simulink library "eltreclib"  (R2017a)
settings: Solver=VariableStepAuto  StartTime=0.0  StopTime=10.0  RelTol=1e-3
libraries: powerlib x46
settings Model: Creator=mayartmal  LastModifiedBy=OspanbekovBK

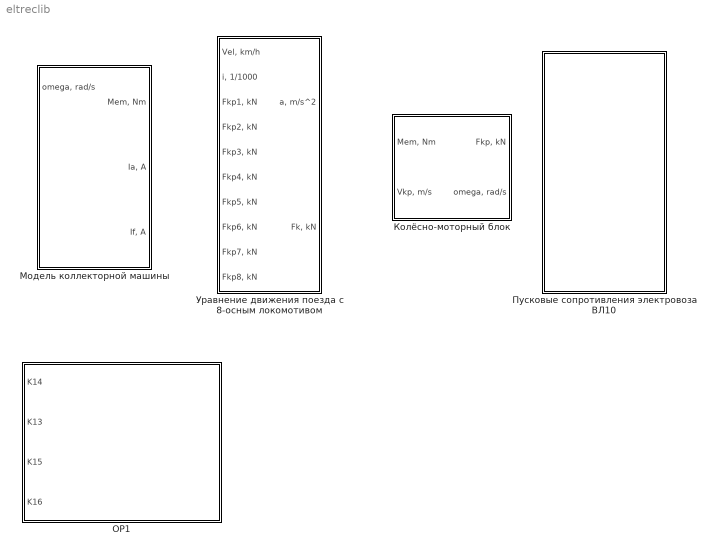
== system eltreclib ==
  OP1 : Subsystem
      mask DialogControl DescTextVar Prompt: Резисторы ослабления поля
  Колёсно-моторный блок : Subsystem  mask{Db=0, mu=0}
      mask prompts: Db "Диаметр бандажа, м"; mu "Передаточное отношение редуктора"
      mask DialogControl DescTextVar Prompt: Здесь можно вписать описание, формулы и другую полезную информацию
  Модель коллекторной машины : Subsystem  mask{Rf=0, Lf=0, Ra=0, La=0, Ce=0, Cm=0, A=0, B=0}
      mask prompts: Rf "Активное сопротивление обмотки возбуждения, Ом"; Lf "Индуктивность обмотки возбуждения, Гн"; Ra "Активное сопротивление обмотки якоря, Ом"; La "Индуктивность обмотки якоря, Гн"; Ce "Константа Ce"; Cm "Константа Cm"; A "Коэффициент A"; B "Коэффициент B"
      mask DialogControl DescTextVar Prompt: Здесь можно вписать описание, формулы и другую полезную информацию
  Пусковые сопротивления электровоза ВЛ10 : Subsystem
  Уравнение движения поезда c 8-осным локомотивом : Subsystem  mask{a0=0, a1=0, a2=0, P=0, Q=0}
      mask prompts: a0 "Коэффициент a0"; a1 "Коэффициент a1"; a2 "Коэффициент a2"; P "Масса локомотива, т"; Q "Масса состава, т"
      mask DialogControl DescTextVar Prompt: Здесь можно вписать описание, формулы и другую полезную информацию

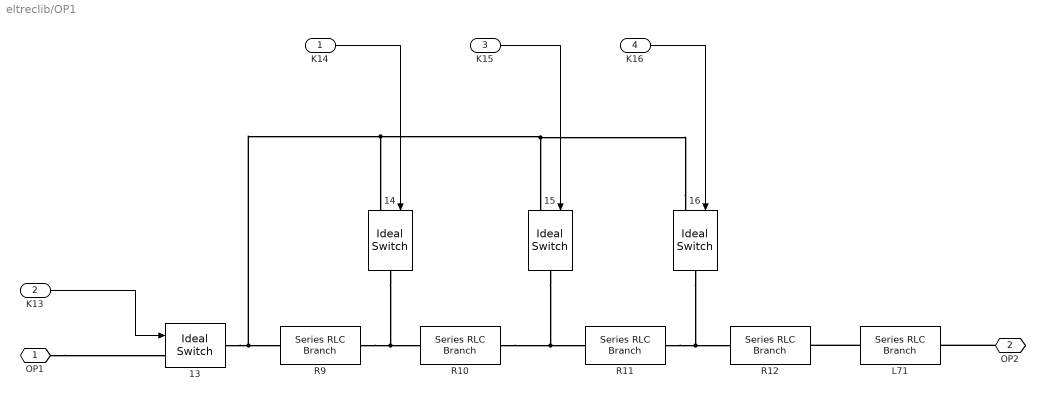
== system eltreclib/OP1 ==
  K14 : Inport
  K13 : Inport  Port=2
  K15 : Inport  Port=3
  K16 : Inport  Port=4
  {13..16} (4 alike) : powerlib/Power Electronics/Ideal Switch  Ron=0.001  Lon=0  IC=0  Rs=1e6  Cs=inf  Measurements=off
  L71 : powerlib/Elements/Series RLC Branch  LConnTagsString=__new0  RConnTagsString=__new0  BranchType=RL  Resistance=0.0236  Inductance=4.5e-3  SetiL0=off  InitialCurrent=0  Capacitance=1e-6  Setx0=off  InitialVoltage=0  Measurements=None
  R10 : powerlib/Elements/Series RLC Branch  LConnTagsString=__new0  RConnTagsString=__new0  BranchType=R  Resistance=0.04  Inductance=1e-3  SetiL0=off  InitialCurrent=0  Capacitance=1e-6  Setx0=off  InitialVoltage=0  Measurements=None
  R11 : powerlib/Elements/Series RLC Branch  LConnTagsString=__new0  RConnTagsString=__new0  BranchType=R  Resistance=0.0222  Inductance=1e-3  SetiL0=off  InitialCurrent=0  Capacitance=1e-6  Setx0=off  InitialVoltage=0  Measurements=None
  R12 : powerlib/Elements/Series RLC Branch  LConnTagsString=__new0  RConnTagsString=__new0  BranchType=R  Resistance=0.01  Inductance=1e-3  SetiL0=off  InitialCurrent=0  Capacitance=1e-6  Setx0=off  InitialVoltage=0  Measurements=None
  R9 : powerlib/Elements/Series RLC Branch  LConnTagsString=__new0  RConnTagsString=__new0  BranchType=R  Resistance=0.1407  Inductance=1e-3  SetiL0=off  InitialCurrent=0  Capacitance=1e-6  Setx0=off  InitialVoltage=0  Measurements=None
  OP1 : PMIOPort  Port=1  Side=Right
  OP2 : PMIOPort  Port=2  Side=Right
  wires:
  K16/1 -> 16/1
  K15/1 -> 15/1
  K13/1 -> 13/1
  K14/1 -> 14/1
  connections:
  OP2/RConn1 -- L71/RConn1
  L71/LConn1 -- R12/RConn1
  OP1/RConn1 -- 13/LConn1
  16/LConn1 -- 14/LConn1 -- 13/RConn1 -- R9/LConn1 -- 15/LConn1
  16/RConn1 -- R11/RConn1 -- R12/LConn1
  15/RConn1 -- R10/RConn1 -- R11/LConn1
  14/RConn1 -- R9/RConn1 -- R10/LConn1

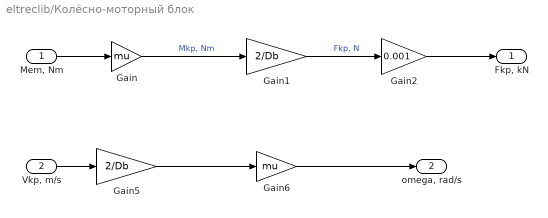
== system eltreclib/Колёсно-моторный блок ==
  "Mem, Nm" : Inport
  "Vkp, m/s" : Inport  Port=2
  Gain : Gain  Gain=mu
  Gain1 : Gain  Gain=2/Db
  Gain2 : Gain  Gain=0.001
  Gain5 : Gain  Gain=2/Db
  Gain6 : Gain  Gain=mu
  "Fkp, kN" : Outport
  "omega, rad/s" : Outport  Port=2
  wires:
  Gain/1 -> Gain1/1  "Mkp, Nm"
  "Mem, Nm"/1 -> Gain/1
  Gain1/1 -> Gain2/1  "Fkp, N"
  Gain5/1 -> Gain6/1
  "Vkp, m/s"/1 -> Gain5/1
  Gain6/1 -> "omega, rad/s"/1
  Gain2/1 -> "Fkp, kN"/1

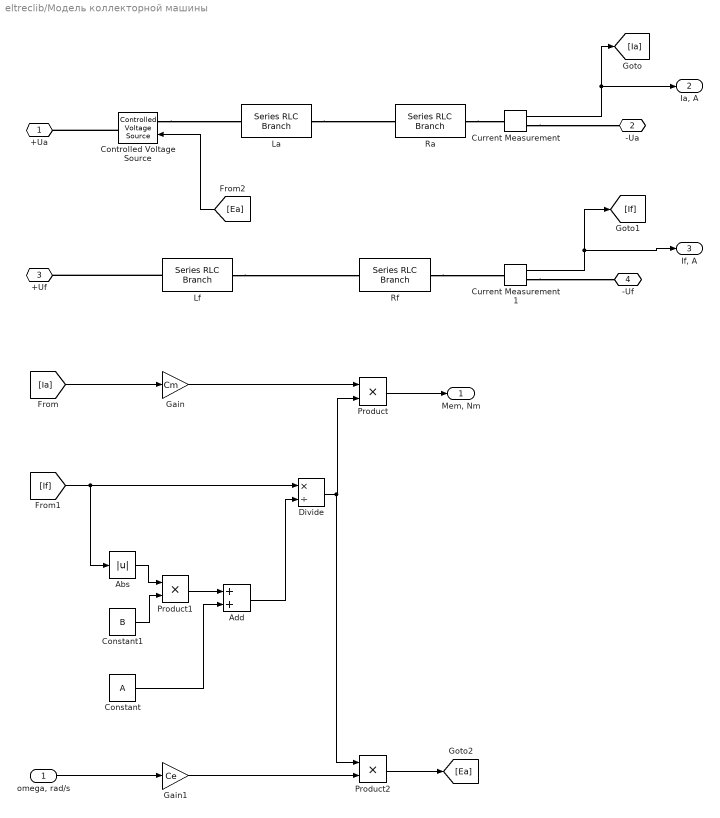
== system eltreclib/Модель коллекторной машины ==
  "omega, rad/s" : Inport
  Abs : Abs
  Add : Sum
  Constant : Constant  Value=A
  Constant1 : Constant  Value=B
  Controlled Voltage Source : powerlib/Electrical Sources/Controlled Voltage Source  Initialize=on  Source_Type=AC  Amplitude=0  Phase=0  Frequency=0  Measurements=None
  Current Measurement : powerlib/Measurements/Current Measurement  PhasorSimulation=off  OutputType=Complex  PSBequivalent=0
  Current Measurement1 : powerlib/Measurements/Current Measurement  PhasorSimulation=off  OutputType=Complex  PSBequivalent=0
  Divide : Product  Inputs=*/
  Gain : Gain  Gain=Cm
  Gain1 : Gain  Gain=Ce
  La : powerlib/Elements/Series RLC Branch  LConnTagsString=__new0  RConnTagsString=__new0  BranchType=L  Resistance=1  Inductance=La  SetiL0=off  InitialCurrent=0  Capacitance=1e-6  Setx0=off  InitialVoltage=0  Measurements=None
  Lf : powerlib/Elements/Series RLC Branch  LConnTagsString=__new0  RConnTagsString=__new0  BranchType=L  Resistance=1  Inductance=Lf  SetiL0=off  InitialCurrent=0  Capacitance=1e-6  Setx0=off  InitialVoltage=0  Measurements=None
  Product : Product
  Product1 : Product
  Product2 : Product
  Ra : powerlib/Elements/Series RLC Branch  LConnTagsString=__new0  RConnTagsString=__new0  BranchType=R  Resistance=Ra  Inductance=1e-3  SetiL0=off  InitialCurrent=0  Capacitance=1e-6  Setx0=off  InitialVoltage=0  Measurements=None
  Rf : powerlib/Elements/Series RLC Branch  LConnTagsString=__new0  RConnTagsString=__new0  BranchType=R  Resistance=Rf  Inductance=1e-3  SetiL0=off  InitialCurrent=0  Capacitance=1e-6  Setx0=off  InitialVoltage=0  Measurements=None
  +Ua : PMIOPort  Port=1  Side=Left
  -Ua : PMIOPort  Port=2  Side=Left
  +Uf : PMIOPort  Port=3  Side=Left
  -Uf : PMIOPort  Port=4  Side=Left
  "Mem, Nm" : Outport
  "Ia, A" : Outport  Port=2
  "If, A" : Outport  Port=3
  wires:
  Product/1 -> "Mem, Nm"/1
  Product2/1 -> [Ea]
  Gain1/1 -> Product2/2
  "omega, rad/s"/1 -> Gain1/1
  Divide/1 -> Product/2, Product2/1
  Add/1 -> Divide/2
  Product1/1 -> Add/1
  Constant/1 -> Add/2
  Constant1/1 -> Product1/2
  Abs/1 -> Product1/1
  [If] -> Abs/1, Divide/1
  Gain/1 -> Product/1
  [Ia] -> Gain/1
  Current Measurement1/1 -> [If], "If, A"/1
  Current Measurement/1 -> "Ia, A"/1, [Ia]
  [Ea] -> Controlled Voltage Source/1
  connections:
  Current Measurement1/RConn1 -- -Uf/RConn1
  Rf/RConn1 -- Current Measurement1/LConn1
  Current Measurement/RConn1 -- -Ua/RConn1
  Ra/RConn1 -- Current Measurement/LConn1
  Controlled Voltage Source/LConn1 -- La/LConn1
  Lf/RConn1 -- Rf/LConn1
  Controlled Voltage Source/RConn1 -- +Ua/RConn1
  Lf/LConn1 -- +Uf/RConn1
  La/RConn1 -- Ra/LConn1

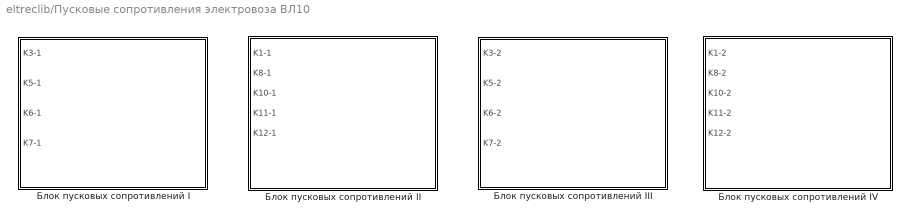
== system eltreclib/Пусковые сопротивления электровоза ВЛ10 ==
  Блок пусковых сопротивлений I : Subsystem
      mask DialogControl DescGroupVar Prompt: Блок пусковых сопротивлений I
      mask DialogControl DescTextVar Prompt: Моделирует схему блока пусковых сопротивлений, собранного из резисторов R1=3.15 Ом, R2=1.47 Ом, R3=1.2 Ом
  Блок пусковых сопротивлений II : Subsystem
      mask DialogControl DescGroupVar Prompt: Блок пусковых сопротивлений II
      mask DialogControl DescTextVar Prompt: Моделирует схему блока пусковых сопротивлений, собранного из резисторов R5=4.725 Ом, R6=0.841 Ом, R7=1.312 Ом
  Блок пусковых сопротивлений III : Subsystem
      mask DialogControl DescGroupVar Prompt: Блок пусковых сопротивлений III
      mask DialogControl DescTextVar Prompt: Моделирует схему блока пусковых сопротивлений, собранного из резисторов R23=1.9425 Ом, R24=0.8 Ом, R25=0.61 Ом
  Блок пусковых сопротивлений IV : Subsystem
      mask DialogControl DescGroupVar Prompt: Блок пусковых сопротивлений IV
      mask DialogControl DescTextVar Prompt: Моделирует схему блока пусковых сопротивлений, собранного из резисторов R27=5.775 Ом, R28=0.595 Ом, R29=0.4315 Ом

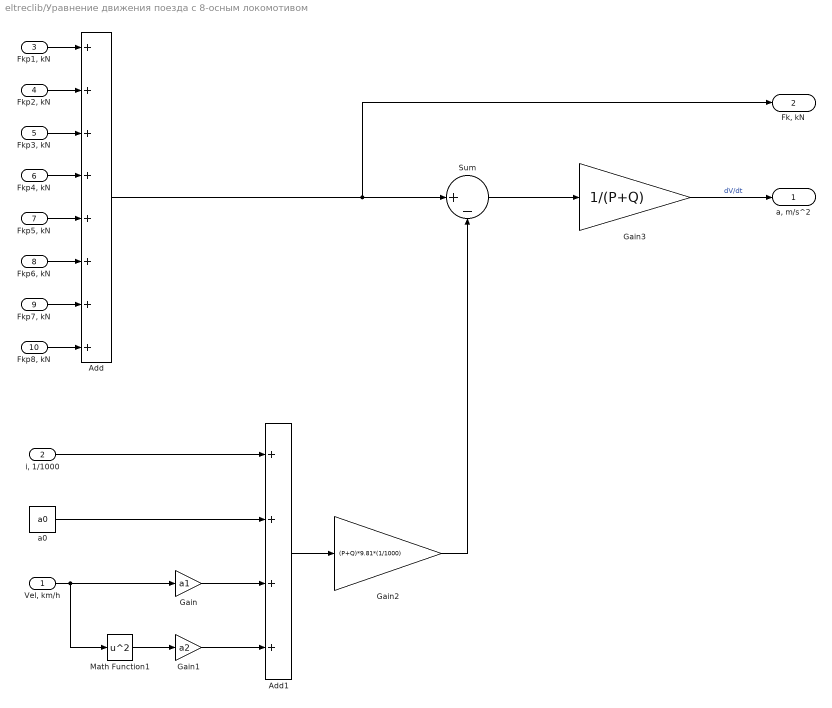
== system eltreclib/Уравнение движения поезда c 8-осным локомотивом ==
  "Vel, km/h" : Inport
  "i, 1/1000" : Inport  Port=2
  "Fkp1, kN" : Inport  Port=3
  "Fkp2, kN" : Inport  Port=4
  "Fkp3, kN" : Inport  Port=5
  "Fkp4, kN" : Inport  Port=6
  "Fkp5, kN" : Inport  Port=7
  "Fkp6, kN" : Inport  Port=8
  "Fkp7, kN" : Inport  Port=9
  "Fkp8, kN" : Inport  Port=10
  Add : Sum  Inputs=++++++++
  Add1 : Sum  Inputs=++++
  Gain : Gain  Gain=a1
  Gain1 : Gain  Gain=a2
  Gain2 : Gain  Gain=(P+Q)*9.81*(1/1000)
  Gain3 : Gain  Gain=1/(P+Q)
  Math Function1 : Math  Operator=square  SaturateOnIntegerOverflow=on
  Sum : Sum  Inputs=|+-
  a0 : Constant  Value=a0
  "a, m/s^2" : Outport
  "Fk, kN" : Outport  Port=2
  wires:
  Add/1 -> "Fk, kN"/1, Sum/1
  "Vel, km/h"/1 -> Math Function1/1, Gain/1
  a0/1 -> Add1/2
  Gain/1 -> Add1/3
  Sum/1 -> Gain3/1
  Gain3/1 -> "a, m/s^2"/1  "dV/dt"
  Gain2/1 -> Sum/2
  Math Function1/1 -> Gain1/1
  Gain1/1 -> Add1/4
  Add1/1 -> Gain2/1
  "Fkp7, kN"/1 -> Add/7
  "Fkp4, kN"/1 -> Add/4
  "Fkp8, kN"/1 -> Add/8
  "Fkp5, kN"/1 -> Add/5
  "Fkp6, kN"/1 -> Add/6
  "Fkp1, kN"/1 -> Add/1
  "Fkp3, kN"/1 -> Add/3
  "Fkp2, kN"/1 -> Add/2
  "i, 1/1000"/1 -> Add1/1

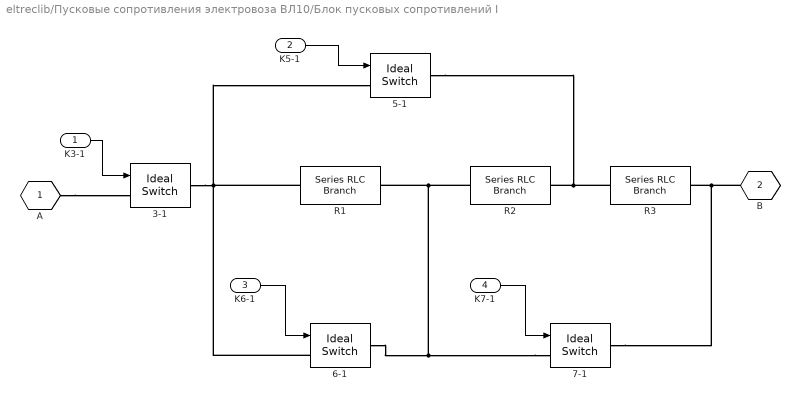
== system eltreclib/Пусковые сопротивления электровоза ВЛ10/Блок пусковых сопротивлений I ==
  K3-1 : Inport
  K5-1 : Inport  Port=2
  K6-1 : Inport  Port=3
  K7-1 : Inport  Port=4
  3-1 : powerlib/Power Electronics/Ideal Switch  Ron=0.001  Lon=0  IC=0  Rs=1e6  Cs=inf  Measurements=off
  5-1 : powerlib/Power Electronics/Ideal Switch  Ron=0.001  Lon=0  IC=0  Rs=1e6  Cs=inf  Measurements=off
  6-1 : powerlib/Power Electronics/Ideal Switch  Ron=0.001  Lon=0  IC=0  Rs=1e6  Cs=inf  Measurements=off
  7-1 : powerlib/Power Electronics/Ideal Switch  Ron=0.001  Lon=0  IC=0  Rs=1e6  Cs=inf  Measurements=off
  R1 : powerlib/Elements/Series RLC Branch  LConnTagsString=__new0  RConnTagsString=__new0  BranchType=R  Resistance=3.15  Inductance=1e-3  SetiL0=off  InitialCurrent=0  Capacitance=1e-6  Setx0=off  InitialVoltage=0  Measurements=None
  R2 : powerlib/Elements/Series RLC Branch  LConnTagsString=__new0  RConnTagsString=__new0  BranchType=R  Resistance=1.47  Inductance=1e-3  SetiL0=off  InitialCurrent=0  Capacitance=1e-6  Setx0=off  InitialVoltage=0  Measurements=None
  R3 : powerlib/Elements/Series RLC Branch  LConnTagsString=__new0  RConnTagsString=__new0  BranchType=R  Resistance=1.2  Inductance=1e-3  SetiL0=off  InitialCurrent=0  Capacitance=1e-6  Setx0=off  InitialVoltage=0  Measurements=None
  A : PMIOPort  Tag=PMCPort  Port=1  Side=Left
  B : PMIOPort  Tag=PMCPort  Port=2  Side=Right
  wires:
  K6-1/1 -> 6-1/1
  K3-1/1 -> 3-1/1
  K7-1/1 -> 7-1/1
  K5-1/1 -> 5-1/1
  connections:
  A/RConn1 -- 3-1/LConn1
  6-1/LConn1 -- R1/LConn1 -- 3-1/RConn1 -- 5-1/LConn1
  R3/LConn1 -- R2/RConn1 -- 5-1/RConn1
  B/RConn1 -- R3/RConn1 -- 7-1/RConn1
  7-1/LConn1 -- 6-1/RConn1 -- R2/LConn1 -- R1/RConn1

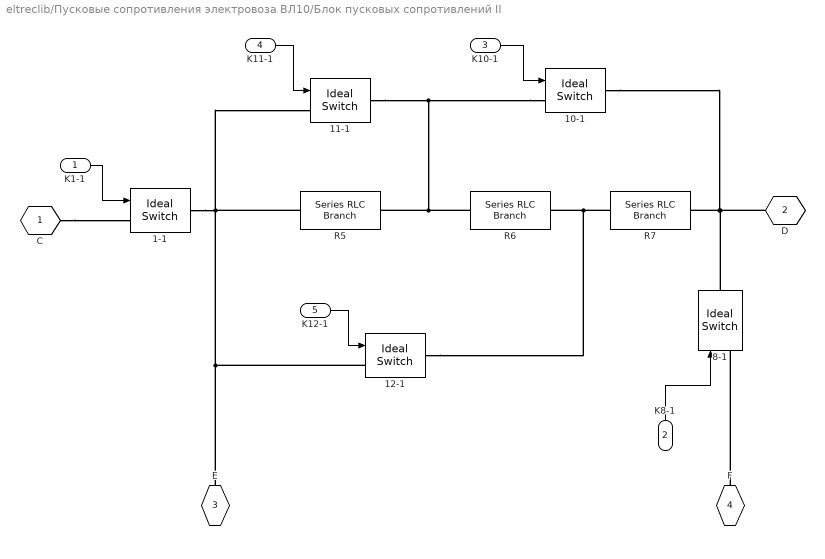
== system eltreclib/Пусковые сопротивления электровоза ВЛ10/Блок пусковых сопротивлений II ==
  K1-1 : Inport
  K8-1 : Inport  Port=2
  K10-1 : Inport  Port=3
  K11-1 : Inport  Port=4
  K12-1 : Inport  Port=5
  1-1 : powerlib/Power Electronics/Ideal Switch  Ron=0.001  Lon=0  IC=0  Rs=1e6  Cs=inf  Measurements=off
  10-1 : powerlib/Power Electronics/Ideal Switch  Ron=0.001  Lon=0  IC=0  Rs=1e6  Cs=inf  Measurements=off
  11-1 : powerlib/Power Electronics/Ideal Switch  Ron=0.001  Lon=0  IC=0  Rs=1e6  Cs=inf  Measurements=off
  12-1 : powerlib/Power Electronics/Ideal Switch  Ron=0.001  Lon=0  IC=0  Rs=1e6  Cs=inf  Measurements=off
  8-1 : powerlib/Power Electronics/Ideal Switch  Ron=0.001  Lon=0  IC=0  Rs=1e6  Cs=inf  Measurements=off
  R5 : powerlib/Elements/Series RLC Branch  LConnTagsString=__new0  RConnTagsString=__new0  BranchType=R  Resistance=4.725  Inductance=1e-3  SetiL0=off  InitialCurrent=0  Capacitance=1e-6  Setx0=off  InitialVoltage=0  Measurements=None
  R6 : powerlib/Elements/Series RLC Branch  LConnTagsString=__new0  RConnTagsString=__new0  BranchType=R  Resistance=0.841  Inductance=1e-3  SetiL0=off  InitialCurrent=0  Capacitance=1e-6  Setx0=off  InitialVoltage=0  Measurements=None
  R7 : powerlib/Elements/Series RLC Branch  LConnTagsString=__new0  RConnTagsString=__new0  BranchType=R  Resistance=1.312  Inductance=1e-3  SetiL0=off  InitialCurrent=0  Capacitance=1e-6  Setx0=off  InitialVoltage=0  Measurements=None
  C : PMIOPort  Tag=PMCPort  Port=1  Side=Left
  D : PMIOPort  Tag=PMCPort  Port=2  Side=Right
  E : PMIOPort  Tag=PMCPort  Port=3  Side=Left
  F : PMIOPort  Tag=PMCPort  Port=4  Side=Right
  wires:
  K8-1/1 -> 8-1/1
  K11-1/1 -> 11-1/1
  K10-1/1 -> 10-1/1
  K1-1/1 -> 1-1/1
  K12-1/1 -> 12-1/1
  connections:
  F/RConn1 -- 8-1/LConn1
  10-1/LConn1 -- 11-1/RConn1 -- R5/RConn1 -- R6/LConn1
  D/RConn1 -- 8-1/RConn1 -- R7/RConn1 -- 10-1/RConn1
  12-1/RConn1 -- R7/LConn1 -- R6/RConn1
  12-1/LConn1 -- E/RConn1 -- R5/LConn1 -- 11-1/LConn1 -- 1-1/RConn1
  C/RConn1 -- 1-1/LConn1

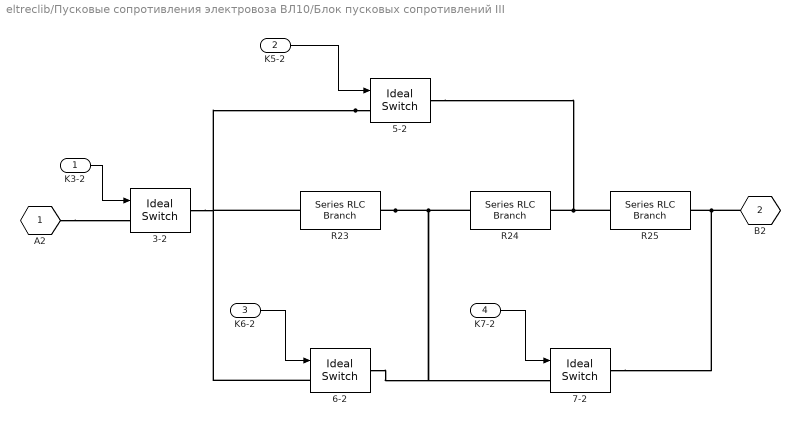
== system eltreclib/Пусковые сопротивления электровоза ВЛ10/Блок пусковых сопротивлений III ==
  K3-2 : Inport
  K5-2 : Inport  Port=2
  K6-2 : Inport  Port=3
  K7-2 : Inport  Port=4
  3-2 : powerlib/Power Electronics/Ideal Switch  Ron=0.001  Lon=0  IC=0  Rs=1e6  Cs=inf  Measurements=off
  5-2 : powerlib/Power Electronics/Ideal Switch  Ron=0.001  Lon=0  IC=0  Rs=1e6  Cs=inf  Measurements=off
  6-2 : powerlib/Power Electronics/Ideal Switch  Ron=0.001  Lon=0  IC=0  Rs=1e6  Cs=inf  Measurements=off
  7-2 : powerlib/Power Electronics/Ideal Switch  Ron=0.001  Lon=0  IC=0  Rs=1e6  Cs=inf  Measurements=off
  R23 : powerlib/Elements/Series RLC Branch  LConnTagsString=__new0  RConnTagsString=__new0  BranchType=R  Resistance=1.9425  Inductance=1e-3  SetiL0=off  InitialCurrent=0  Capacitance=1e-6  Setx0=off  InitialVoltage=0  Measurements=None
  R24 : powerlib/Elements/Series RLC Branch  LConnTagsString=__new0  RConnTagsString=__new0  BranchType=R  Resistance=0.8  Inductance=1e-3  SetiL0=off  InitialCurrent=0  Capacitance=1e-6  Setx0=off  InitialVoltage=0  Measurements=None
  R25 : powerlib/Elements/Series RLC Branch  LConnTagsString=__new0  RConnTagsString=__new0  BranchType=R  Resistance=0.61  Inductance=1e-3  SetiL0=off  InitialCurrent=0  Capacitance=1e-6  Setx0=off  InitialVoltage=0  Measurements=None
  A2 : PMIOPort  Tag=PMCPort  Port=1  Side=Left
  B2 : PMIOPort  Tag=PMCPort  Port=2  Side=Right
  wires:
  K5-2/1 -> 5-2/1
  K7-2/1 -> 7-2/1
  K3-2/1 -> 3-2/1
  K6-2/1 -> 6-2/1
  connections:
  R23/RConn1 -- R24/LConn1 -- 6-2/RConn1 -- 7-2/LConn1
  7-2/RConn1 -- R25/RConn1 -- B2/RConn1
  5-2/RConn1 -- R24/RConn1 -- R25/LConn1
  5-2/LConn1 -- 3-2/RConn1 -- R23/LConn1 -- 6-2/LConn1
  A2/RConn1 -- 3-2/LConn1

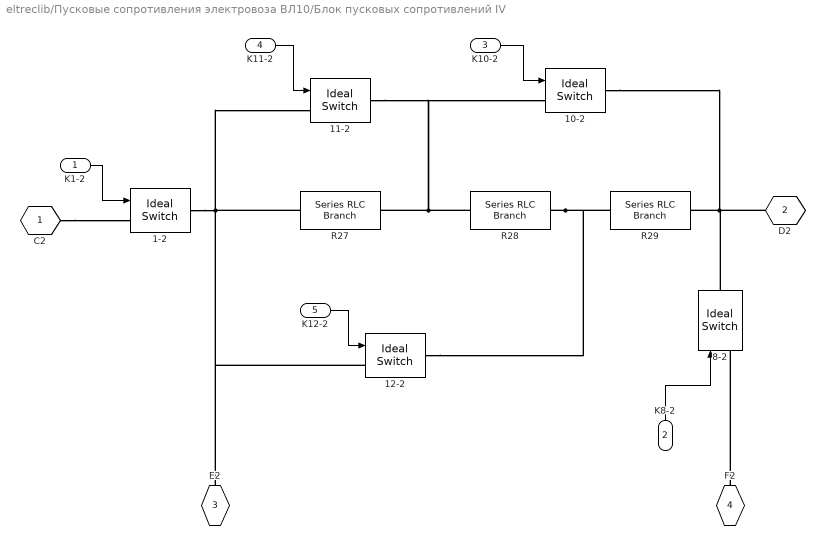
== system eltreclib/Пусковые сопротивления электровоза ВЛ10/Блок пусковых сопротивлений IV ==
  K1-2 : Inport
  K8-2 : Inport  Port=2
  K10-2 : Inport  Port=3
  K11-2 : Inport  Port=4
  K12-2 : Inport  Port=5
  1-2 : powerlib/Power Electronics/Ideal Switch  Ron=0.001  Lon=0  IC=0  Rs=1e6  Cs=inf  Measurements=off
  10-2 : powerlib/Power Electronics/Ideal Switch  Ron=0.001  Lon=0  IC=0  Rs=1e6  Cs=inf  Measurements=off
  11-2 : powerlib/Power Electronics/Ideal Switch  Ron=0.001  Lon=0  IC=0  Rs=1e6  Cs=inf  Measurements=off
  12-2 : powerlib/Power Electronics/Ideal Switch  Ron=0.001  Lon=0  IC=0  Rs=1e6  Cs=inf  Measurements=off
  8-2 : powerlib/Power Electronics/Ideal Switch  Ron=0.001  Lon=0  IC=0  Rs=1e6  Cs=inf  Measurements=off
  R27 : powerlib/Elements/Series RLC Branch  LConnTagsString=__new0  RConnTagsString=__new0  BranchType=R  Resistance=5.775  Inductance=1e-3  SetiL0=off  InitialCurrent=0  Capacitance=1e-6  Setx0=off  InitialVoltage=0  Measurements=None
  R28 : powerlib/Elements/Series RLC Branch  LConnTagsString=__new0  RConnTagsString=__new0  BranchType=R  Resistance=0.595  Inductance=1e-3  SetiL0=off  InitialCurrent=0  Capacitance=1e-6  Setx0=off  InitialVoltage=0  Measurements=None
  R29 : powerlib/Elements/Series RLC Branch  LConnTagsString=__new0  RConnTagsString=__new0  BranchType=R  Resistance=0.4315  Inductance=1e-3  SetiL0=off  InitialCurrent=0  Capacitance=1e-6  Setx0=off  InitialVoltage=0  Measurements=None
  C2 : PMIOPort  Tag=PMCPort  Port=1  Side=Left
  D2 : PMIOPort  Tag=PMCPort  Port=2  Side=Right
  E2 : PMIOPort  Tag=PMCPort  Port=3  Side=Left
  F2 : PMIOPort  Tag=PMCPort  Port=4  Side=Right
  wires:
  K12-2/1 -> 12-2/1
  K1-2/1 -> 1-2/1
  K10-2/1 -> 10-2/1
  K11-2/1 -> 11-2/1
  K8-2/1 -> 8-2/1
  connections:
  C2/RConn1 -- 1-2/LConn1
  1-2/RConn1 -- 11-2/LConn1 -- R27/LConn1 -- E2/RConn1 -- 12-2/LConn1
  R28/RConn1 -- R29/LConn1 -- 12-2/RConn1
  10-2/RConn1 -- R29/RConn1 -- 8-2/RConn1 -- D2/RConn1
  R28/LConn1 -- R27/RConn1 -- 11-2/RConn1 -- 10-2/LConn1
  F2/RConn1 -- 8-2/LConn1
